simulink model "Anim"  (R2025b)
settings: Solver=VariableStepAuto  StartTime=0.0  StopTime=30  RelTol=1e-3
libraries: sim3dlib x5
settings Model: Creator=admin  LastModifiedBy=admin

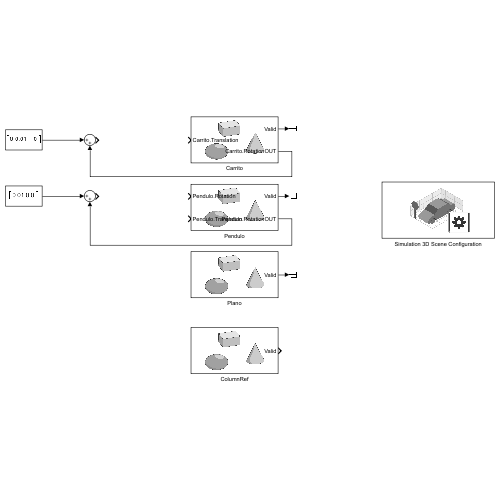
[thumbnail: Simulink's stored preview of the top-level diagram]
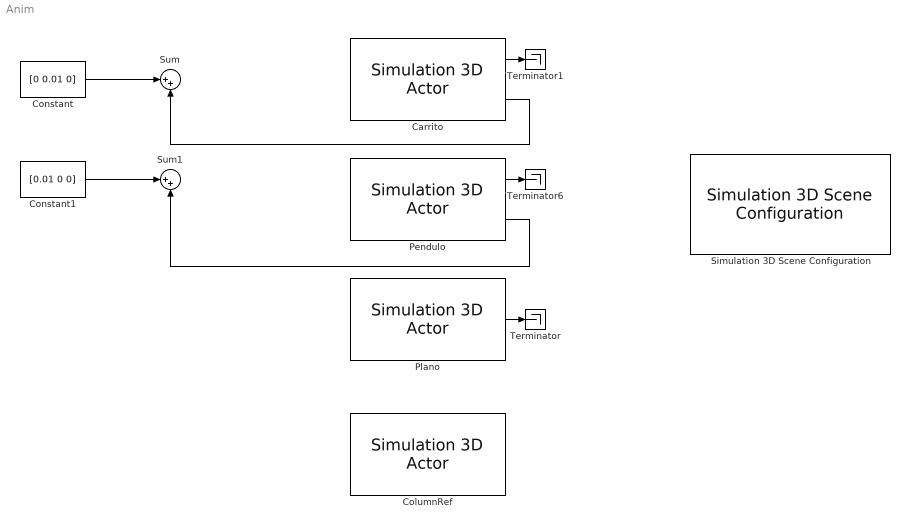
== system Anim ==
  Carrito : sim3dlib/Simulation 3D Actor  Priority=1  ActorName=Carrito  ParentName=Scene Origin  Operation=Create at setup  InitScriptText=|  SampleTime=-1  Translation=[0 0 0]  Rotation=[0 0 0]  Scale=[1 1 1]  InputsText=Carrito.Translation  OutputsText=Carrito.Rotation  aMode=5  ActorTag=Carrito  ActorType=Sim3dActor  ID=C
      | createShape(Actor, 'box', [0.05 0.1 0.05]);
      | Actor.Color = [1 0 0];
      | Actor.Translation = [0 0 0];
      | Actor.Scale = [1 1 1];
      | Actor.Physics = false;
      | Actor.Gravity = false;
      | 
      | % Create Axis Arrows
  ColumnRef : sim3dlib/Simulation 3D Actor  Priority=1  ActorName=Sim3dActor1  ParentName=Scene Origin  Operation=Create at setup  InitScriptText=|  SampleTime=-1  Translation=[0.1 0 0.1]  Rotation=[0 0 0]  Scale=[1 1 1]  aMode=5  ActorTag=Sim3dActor1  ActorType=Sim3dActor  ID=1
      | createShape(Actor, 'cylinder', [0.02 0.02 0.2]);
      | Actor.Color = [1 0 0];
      | Actor.Color = [1 1 1];
      | Actor.Translation = [0.1 0 0.1];
      | Actor.Rotation = [0 0 0];
      | Actor.Scale = [1 1 1];
      | Actor.Physics = false;
      | Actor.Gravity = false;
      | 
      | % Create Axis Arrows
  Constant : Constant  Value=[0 0.01 0]
  Constant1 : Constant  Value=[0.01 0 0]
  Pendulo : sim3dlib/Simulation 3D Actor  Priority=1  ActorName=Pendulo  ParentName=Carrito  Operation=Create at setup  InitScriptText=|  SampleTime=-1  Translation=[0 0 0.06]  Rotation=[0 0 0]  Scale=[1 1 1]  InputsText="Pendulo.Rotation    Pendulo.Translation"  OutputsText=Pendulo.Rotation  aMode=5  ActorTag=Pendulo  ActorType=Sim3dActor  ID=C
      | createShape(Actor, 'cylinder', [0.01 0.01 0.2]);Actor.Color = [1 0 0];
      | Actor.Color = [0 0 1];
      | Actor.Translation = [0 0 0.06];
      | Actor.Scale = [1 1 1];
      | Actor.Physics = false;
      | Actor.Gravity = false;
  Plano : sim3dlib/Simulation 3D Actor  Priority=1  ActorName=Sim3dActor2  ParentName=Scene Origin  Operation=Create at setup  InitScriptText=|  SampleTime=-1  Translation=[0 0 0]  Rotation=[0 0 0]  Scale=[1 1 1]  aMode=5  ActorTag=Sim3dActor2  ActorType=Sim3dActor  ID=2
      | createShape(Actor, 'plane', [5 5 0.1]);
      | Actor.PreciseContacts = true;
      | Actor.Color = [0 0 0];
  Simulation 3D Scene Configuration : sim3dlib/Simulation 3D Scene Configuration  Priority=0  ProjectFormat=Default Scenes  SceneDesc=Empty scene  ProjectName=C:\Program Files\MATLAB\R2025b\toolbox\shared\sim3d_projects\automotive_project_windows\UE\WindowsNoEditor\VehicleSimulation.exe  ScenePath=/Game/Maps/HwStrght  EnableOpenDRIVE=off  vehTagList={'Carrito';'Custom';'Pendulo';'Scene Origin';'Sim3dActor1';'Sim3dActor2'}  vehTag=Scene Origin  AttachedCameraRelativeTranslation=[-0.75 0 0.25]  FreeCameraDefaultInitialTranslation=[-6, 0, 2]  AttachedCameraRelativeRotation=[0 -25 0]  FreeCameraDefaultInitialRotation=[0, -15, 0]  ViewpointName=Custom  FreeCameraInitialTranslation=[0, 0, 0]  ViewpointTranslation=[0 0 0]  FreeCameraInitialRotation=[0, 0, 0]  ViewpointRotation=[0 0 0]  OpVisEn=off  Ts=.02  EnableWindow=on  EnableRemoteAccess=off  EnableWeather=off  SunAzimuth=90  SunAltitude=40.0  EnableGeospatialSun=off  Latitude=0  Longitude=0  Date=2023-01-01  Time=10:30:00  GeoTimeZone=-5.0  SunDaylightSaving=off  wind=1  clouds=10  EnableVolumetricClouds=off  CloudCoverage=0  CloudAltitude=6  fog=0  rain=0  RaindropsEffect=off  SnowDensity=0  EnableGeospatial=off  TilesetSource=Earth terrain  UseTrueOrigin=off  OriginHeight=200  OriginLatitude=40.744652  OriginLongitude=-73.988864  MapStyle=Aerial  AdditionalAssetIDs=[]  UseAdvancedSunSky=off  SolarTime=11  TimeZone=-5  Day=21  Month=9  Year=2022  UseDaylightSavingTime=on  DSTStartDay=10  DSTStartMonth=3  DSTEndDay=3  DSTEndMonth=11  DSTSwitchHour=2  sensorTag=MainCamera1  sensorId=1  sensorName=MainCamera1  mountLoc=Origin  offsetFlag=off  tmountOffset=[0, 0, 0]  rmountOffset=[0, 0, 0]  HorizontalResolution=1280  VerticalResolution=720  HorizontalFOV=60  mountPoint=[0 0 0]  mountOrientation=[0 0 0]  aMode=5  ID=1  GeoTrigger=Inactive  ViewNameList={'Custom'}  ViewTranslationList={'[0 0 0]'}  ViewRotationList={'[0 0 0]'}
      settings: LibrarySourceBlock=sl3dlib/Simulation 3D/Environment/Simulation 3D Scene Configuration
  Sum : Sum  Inputs=|++
  Sum1 : Sum  Inputs=|++
  Terminator : Terminator
  Terminator1 : Terminator
  Terminator6 : Terminator
  wires:
  Constant/1 -> Sum/1
  Constant1/1 -> Sum1/1
  Carrito/1 -> Terminator1/1
  Plano/1 -> Terminator/1
  Pendulo/1 -> Terminator6/1
  Pendulo/2 -> Sum1/2
  Carrito/2 -> Sum/2
